simulink model "Bicycle_LQR_DiscKappa"  (R2024b)
settings: Solver=ode45  StartTime=0.0  StopTime=150  MaxStep=0.05  RelTol=1e-3
InitFcn:
  | clear persistent_anim_update
  | clear nearest_ref_point
values from neighbouring files (symbols this model uses):
  K_lqr = dlqr(A_d, B_d, Q_lqr, R_lqr)    [LQRScript_DiscKappa.m]
  theta_init = theta_ref_arr(closest_idx)    [LQRScript_DiscKappa.m]
  Ts = 0.02    [LQRScript_DiscKappa.m]
  x_init = sp(1)    [LQRScript_DiscKappa.m]
  y_init = sp(2)    [LQRScript_DiscKappa.m]
settings Model: PacingRate=10  Creator=kasimesen  LastModifiedBy=kasimesen
settings DataIOCC: ReturnWorkspaceOutputs=off

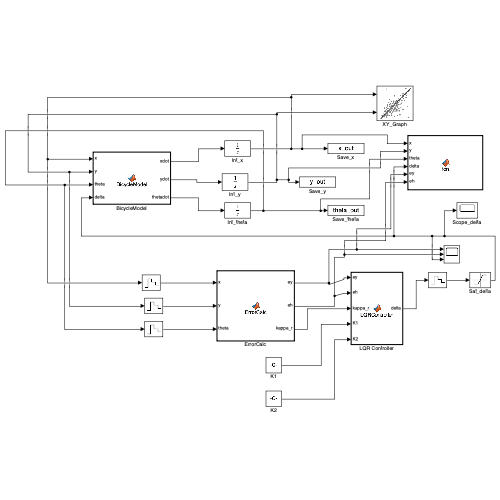
[thumbnail: Simulink's stored preview of the top-level diagram]
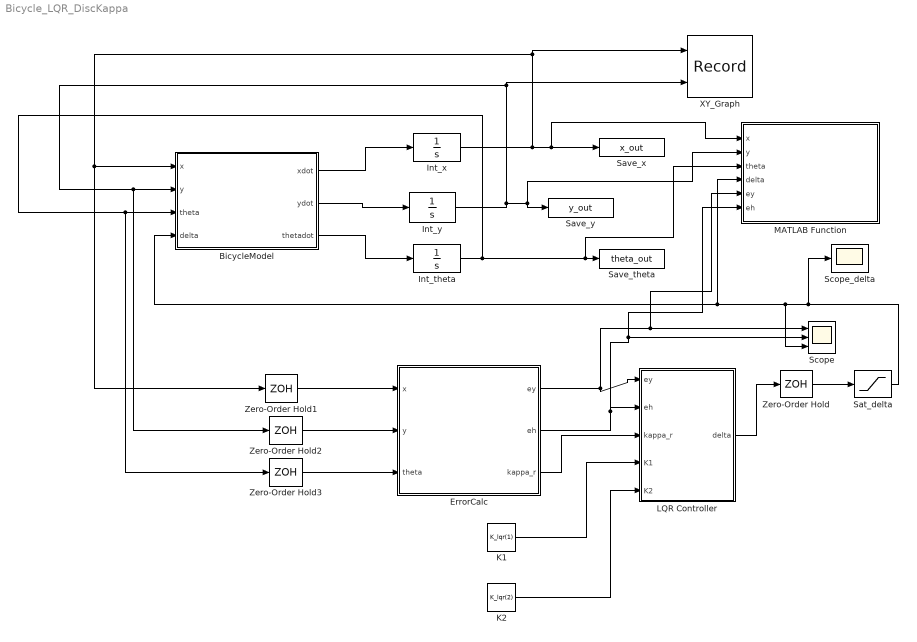
== system Bicycle_LQR_DiscKappa ==
  BicycleModel : MATLAB Function  TreatAsAtomicUnit=on
  ErrorCalc : MATLAB Function  TreatAsAtomicUnit=on
  Int_theta : Integrator  InitialCondition=theta_init
  Int_x : Integrator  InitialCondition=x_init
  Int_y : Integrator  InitialCondition=y_init
  K1 : Constant  Value=K_lqr(1)
  K2 : Constant  Value=K_lqr(2)
  LQR Controller : MATLAB Function  TreatAsAtomicUnit=on
  MATLAB Function : MATLAB Function  TreatAsAtomicUnit=on
  Sat_delta : Saturate  UpperLimit=0.5236  LowerLimit=-0.5236
  Save_theta : ToWorkspace  VariableName=theta_out  SaveFormat=Timeseries  SampleTime=-1
  Save_x : ToWorkspace  VariableName=x_out  SaveFormat=Timeseries  SampleTime=-1
  Save_y : ToWorkspace  VariableName=y_out  SaveFormat=Timeseries  SampleTime=-1
  Scope : Scope  NumInputPorts=3
  Scope_delta : Scope
  XY_Graph : Record  FileSettingsInternal="{\"entries\":[{\"content\":{\"excelSettings\":{\"content\":{},\"type\":\"Streamout.ExcelSettings\"}},\"type\":\"Streamout.FileSettingStorage\",\"uuid\":\"\"}],\"packageUris\":[\"http:\\/\\/schema.mathworks.com\\/mf0\\/streamout_blocks\\/R2020a\"],\"version\":\"1.0\"}"  Layout=[1 1]  SignalsInternal="{\"entries\":[{\"content\":{\"signals\":[{\"content\":{\"blockPath\":[],\"dimensions\":[1],\"domain\":\"\",\"lineColor\":\"#a2142f\",\"plots\":[ 1 ],\"port\":1,\"sid\":[\"\"],\"signalID\":1,\"signalName\":\"Int_x\"},\"type\":\"RecordBlkView.Signal\",\"uuid\":\"\"},{\"content\":{\"blockPath\":[],\"dimensions\":[1],\"domain\":\"\",\"lineColor\":\"#139fff\",\"plots\":[ 1 ],\"port\":2,\"sid\":[\"\"],\"signalID\":2,\"signalName\":\"Int_y\"},\"type\":\"RecordBlkView.Signal\",\"uuid\":\"\"}]},\"type\":\"RecordBlkView.InputSignals\",\"uuid\":\"\"}],\"packageUris\":[\"http:\\/\\/schema.mathworks.com\\/mf0\\/streamout_blocks\\/R2020a\"],\"version\":\"1.0\"}"  VisualizationBindings="{\"xyplotplugin\":{\"info\":[{\"series\":[{\"bindingParametersList\":[{\"parameter\":\"X-Axis\",\"signalID\":1,\"signalName\":\"Int_x\"},{\"parameter\":\"Y-Axis\",\"signalID\":2,\"signalName\":\"Int_y\"}],\"seriesID\":0}],\"subplotID\":1}]}}"  CompatibilityTag=XY
  Zero-Order Hold{,1..3} (4 alike) : ZeroOrderHold  SampleTime=Ts
  wires:
  ErrorCalc/1(ey) -> MATLAB Function/5(ey), Scope/1, LQR Controller/1(ey)
  ErrorCalc/2(eh) -> LQR Controller/2(eh), MATLAB Function/6(eh), Scope/2
  LQR Controller/1(delta) -> Zero-Order Hold/1
  Sat_delta/1 -> Scope/3, MATLAB Function/4(delta), BicycleModel/4(delta), Scope_delta/1
  BicycleModel/1(xdot) -> Int_x/1
  BicycleModel/2(ydot) -> Int_y/1
  BicycleModel/3(thetadot) -> Int_theta/1
  Int_x/1 -> MATLAB Function/1(x), Save_x/1, Zero-Order Hold1/1, BicycleModel/1(x), XY_Graph/1
  Int_y/1 -> Zero-Order Hold2/1, BicycleModel/2(y), XY_Graph/2, Save_y/1, MATLAB Function/2(y)
  Int_theta/1 -> MATLAB Function/3(theta), Save_theta/1, Zero-Order Hold3/1, BicycleModel/3(theta)
  Zero-Order Hold/1 -> Sat_delta/1
  ErrorCalc/3(kappa_r) -> LQR Controller/3(kappa_r)
  K1/1 -> LQR Controller/4(K1)
  K2/1 -> LQR Controller/5(K2)
  Zero-Order Hold1/1 -> ErrorCalc/1(x)
  Zero-Order Hold2/1 -> ErrorCalc/2(y)
  Zero-Order Hold3/1 -> ErrorCalc/3(theta)

== matlab function Bicycle_LQR_DiscKappa/BicycleModel ==
  data: x input; xdot output; y input; theta input; delta input; ydot output; thetadot output
function [xdot, ydot, thetadot] = BicycleModel(x, y, theta, delta)
%
% Girişler: x, y, theta (araç durumu), delta (direksiyon)
% Çıkışlar: xdot, ydot, thetadot

L     = 2.0;    % Dingil mesafesi (m)
lr    = 1.0;    % Arka aks - kütle merkezine uzaklık (m)
v_ref = 8.0;    % Referans hız (m/s)

% Slip angle
beta = atan((lr/L) * tan(delta));

% Kinematik denklemler
xdot     = v_ref * cos(theta + beta);
ydot     = v_ref * sin(theta + beta);
thetadot = (v_ref/L) * cos(beta) * tan(delta);
end

== matlab function Bicycle_LQR_DiscKappa/ErrorCalc ==
  data: x input; ey output; y input; theta input; eh output; kappa_r output
function [ey, eh, kappa_r] = ErrorCalc(x, y, theta)
coder.extrinsic('nearest_ref_point');

xr  = 0;
yr  = 0;
thr = 0;
kappa_r = 0;
[xr, yr, thr, kappa_r] = nearest_ref_point(x, y);

approach_dist = 10.0;

dist = sqrt((x - xr)^2 + (y - yr)^2);

if dist >= approach_dist
    % UZAK
    desired = atan2(yr - y, xr - x);
    ey = 0;
    eh = mod(theta - desired + pi, 2*pi) - pi;
else
    % YAKIN
    dx = x - xr;
    dy = y - yr;
    ey = -sin(thr)*dx + cos(thr)*dy;
    eh = mod(theta - thr + pi, 2*pi) - pi;
end
end

== matlab function Bicycle_LQR_DiscKappa/MATLAB Function ==
  data: x input; y input; theta input; delta input; ey input; eh input
function fcn(x, y, theta, delta, ey, eh)
% ANİMASYON
% Referans yolu workspace'ten okur.

coder.extrinsic('persistent_anim_update');
persistent_anim_update(x, y, theta);
end

== matlab function Bicycle_LQR_DiscKappa/LQR Controller ==
  data: ey input; delta output; eh input; kappa_r input; K1 input; K2 input
function delta = LQRController(ey, eh, kappa_r, K1, K2)
% Girişler: ey, eh, kappa_r
% Çıkış: delta

L = 2.0;

% Feedforward
delta_ff = atan(kappa_r * L);

% Feedback
delta_fb = -K1*ey - K2*eh;

% Toplam
delta = delta_ff + delta_fb;
end
